simulink model "smc"  (R2020a)
settings: Solver=FixedStepAuto  StartTime=0.0  StopTime=tstop  FixedStep=tstep  RelTol=1e-3
values from neighbouring files (symbols this model uses):
  tstep = 0.01    [data.m]
  xic = [-2; 1]    [data.m]
  xmic = [-3; -2]    [data.m]
settings Model: Creator=Maithili Shetty  LastModifiedBy=Maithili Shetty
settings DataIOCC: ReturnWorkspaceOutputs=off

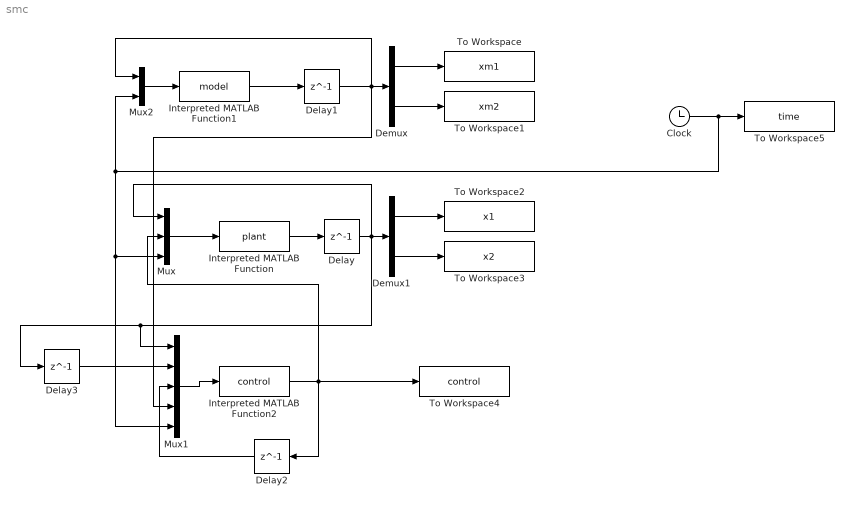
== system smc ==
  Clock : Clock
  Delay : Delay  DelayLength=1  InitialCondition=xic  SampleTime=tstep
  Delay1 : Delay  DelayLength=1  InitialCondition=xmic  SampleTime=tstep
  Delay2 : Delay  DelayLength=1  SampleTime=tstep
  Delay3 : Delay  DelayLength=1  SampleTime=tstep
  Demux : Demux  Outputs=2
  Demux1 : Demux  Outputs=2
  Interpreted MATLAB Function : MATLABFcn  MATLABFcn=plant  OutputDimensions=2
  Interpreted MATLAB Function1 : MATLABFcn  MATLABFcn=model  OutputDimensions=2
  Interpreted MATLAB Function2 : MATLABFcn  MATLABFcn=control  OutputDimensions=1
  Mux : Mux  Inputs=3
  Mux1 : Mux  Inputs=5
  Mux2 : Mux  Inputs=2
  To Workspace : ToWorkspace  VariableName=xm1  SampleTime=-1
  To Workspace1 : ToWorkspace  VariableName=xm2  SampleTime=-1
  To Workspace2 : ToWorkspace  VariableName=x1  SampleTime=-1
  To Workspace3 : ToWorkspace  VariableName=x2  SampleTime=-1
  To Workspace4 : ToWorkspace  VariableName=control  SampleTime=-1
  To Workspace5 : ToWorkspace  VariableName=time  SampleTime=-1
  wires:
  Interpreted MATLAB Function/1 -> Delay/1
  Mux/1 -> Interpreted MATLAB Function/1
  Interpreted MATLAB Function1/1 -> Delay1/1
  Demux/1 -> To Workspace/1
  Demux/2 -> To Workspace1/1
  Demux1/1 -> To Workspace2/1
  Demux1/2 -> To Workspace3/1
  Delay/1 -> Delay3/1, Mux1/1, Mux/1, Demux1/1
  Delay1/1 -> Mux1/4, Mux2/1, Demux/1
  Interpreted MATLAB Function2/1 -> Mux/2, To Workspace4/1, Delay2/1
  Delay3/1 -> Mux1/2
  Mux1/1 -> Interpreted MATLAB Function2/1
  Clock/1 -> Mux1/5, Mux/3, Mux2/2, To Workspace5/1
  Delay2/1 -> Mux1/3
  Mux2/1 -> Interpreted MATLAB Function1/1
